simulink model "Appl_PaAdjustModel"  (R2018b)
settings: configuration reference "CodeConfig_10_ms" (kept outside this file)
undefined symbols (not defined in the file): CAL_HightMotorRunInterval_100ms, CAL_MotorDiffToStart_100ms, CAL_MotorStopTime_50ms, D_Relay_DownBackFault, D_Relay_UpFrontFault, D_ToleranceDistance, enSeatMoveCmd, FALSE, TRUE
libraries: DareLib x84, simulink x2
(part 2 of 3)

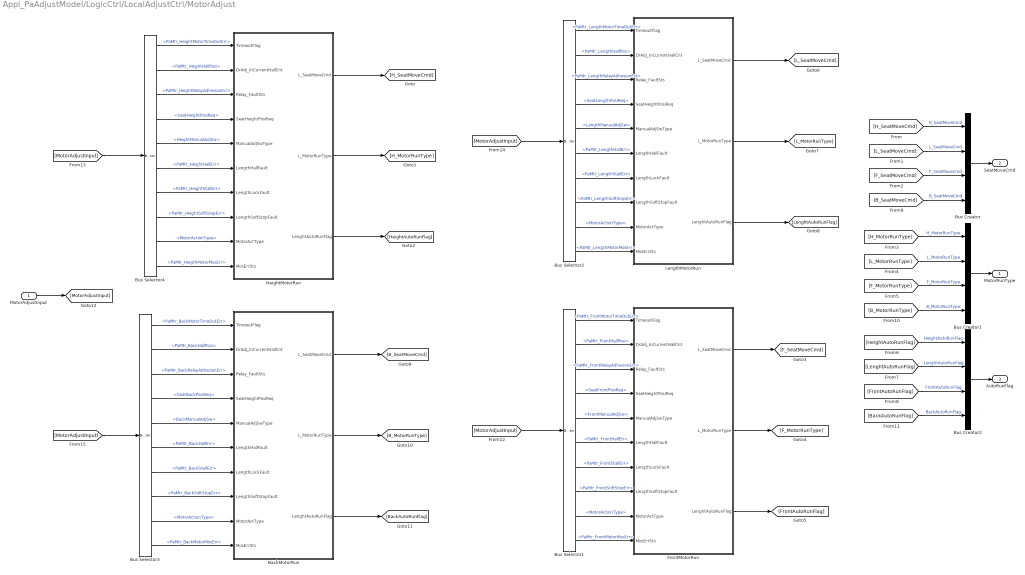
== system Appl_PaAdjustModel/LogicCtrl/LocalAdjustCtrl/MotorAdjust ==
  MotorAdjustInput : Inport
  BackMotorRun : Subsystem
      settings: AttributesFormatString=靠背电机运动状态与处理
  Bus Creator : BusCreator  Inputs=4
  Bus Creator1 : BusCreator  Inputs=4
  Bus Creator2 : BusCreator  Inputs=4
  Bus Selector1 : BusSelector  OutputSignals=RteInputBus.ErrSts.PaMtr_FrontMotorTimeOutErr,RteInputBus.HallCnt.PaMtr_FrontHallPosi,RteInputBus.ErrSts.PaMtr_FrontRelayAdhesionErr,MotorReq.SeatFrontPosiReq,MotorReq.FrontManualAdjSw,RteInputBus.ErrSts.PaMtr_FrontHallErr,RteInputBus.ErrSts.PaMtr_FrontStallErr,RteInputBus.ErrSts.PaMtr_FrontSoftStopErr,MotorReq.MotorActionType,RteInputBus.MosErrSts.PaMtr_FrontMotorMosErr
  Bus Selector2 : BusSelector  OutputSignals=RteInputBus.ErrSts.PaMtr_LengthMotorTimeOutErr,RteInputBus.HallCnt.PaMtr_LengthHallPosi,RteInputBus.ErrSts.PaMtr_LengthRelayAdhesionErr,MotorReq.SeatLengthPosiReq,MotorReq.LengthManualAdjSw,RteInputBus.ErrSts.PaMtr_LengthHallErr,RteInputBus.ErrSts.PaMtr_LengthStallErr,RteInputBus.ErrSts.PaMtr_LengthSoftStopErr,MotorReq.MotorActionType,RteInputBus.MosErrSts.PaMtr_LengthMotorMosErr
  Bus Selector3 : BusSelector  OutputSignals=RteInputBus.ErrSts.PaMtr_BackMotorTimeOutErr,RteInputBus.HallCnt.PaMtr_BackHallPosi,RteInputBus.ErrSts.PaMtr_BackRelayAdhesionErr,MotorReq.SeatBackPosiReq,MotorReq.BackManualAdjSw,RteInputBus.ErrSts.PaMtr_BackHallErr,RteInputBus.ErrSts.PaMtr_BackStallErr,RteInputBus.ErrSts.PaMtr_BackSoftStopErr,MotorReq.MotorActionType,RteInputBus.MosErrSts.PaMtr_BackMotorMosErr
  Bus Selector4 : BusSelector  OutputSignals=RteInputBus.ErrSts.PaMtr_HeightMotorTimeOutErr,RteInputBus.HallCnt.PaMtr_HeightHallPosi,RteInputBus.ErrSts.PaMtr_HeightRelayAdhesionErr,MotorReq.SeatHeightPosiReq,MotorReq.HeightManualAdjSw,RteInputBus.ErrSts.PaMtr_HeightHallErr,RteInputBus.ErrSts.PaMtr_HeightStallErr,RteInputBus.ErrSts.PaMtr_HeightSoftStopErr,MotorReq.MotorActionType,RteInputBus.MosErrSts.PaMtr_HeigthMotorMosErr
  FrontMotorRun : Subsystem
      settings: AttributesFormatString=腿托电机运动状态与处理
  HeightMotorRun : Subsystem
      settings: AttributesFormatString=高度电机运动状态与处理
  LengthMotorRun : Subsystem  Description=纵向电机
      settings: AttributesFormatString=纵向电机运动请求处理
  MotorRunType : Outport
  SeatMoveCmd : Outport  Port=2
  AutoRunFlag : Outport  Port=3
  wires:
  [H_SeatMoveCmd] -> Bus Creator/1  "H_SeatMoveCmd"
  [L_SeatMoveCmd] -> Bus Creator/2  "L_SeatMoveCmd"
  [F_SeatMoveCmd] -> Bus Creator/3  "F_SeatMoveCmd"
  [B_SeatMoveCmd] -> Bus Creator/4  "B_SeatMoveCmd"
  [H_MotorRunType] -> Bus Creator1/1  "H_MotorRunType"
  [L_MotorRunType] -> Bus Creator1/2  "L_MotorRunType"
  [F_MotorRunType] -> Bus Creator1/3  "F_MotorRunType"
  [B_MotorRunType] -> Bus Creator1/4  "B_MotorRunType"
  [LenghtAutoRunFlag] -> Bus Creator2/2  "LenghtAutoRunFlag"
  [HeightAutoRunFlag] -> Bus Creator2/1  "HeightAutoRunFlag"
  [FrontAutoRunFlag] -> Bus Creator2/3  "FrontAutoRunFlag"
  [BackAutoRunFlag] -> Bus Creator2/4  "BackAutoRunFlag"
  Bus Creator/1 -> SeatMoveCmd/1
  Bus Creator1/1 -> MotorRunType/1
  Bus Creator2/1 -> AutoRunFlag/1
  BackMotorRun/3(LenghtAutoRunFlag) -> [BackAutoRunFlag]
  LengthMotorRun/3(LenghtAutoRunFlag) -> [LenghtAutoRunFlag]
  FrontMotorRun/3(LenghtAutoRunFlag) -> [FrontAutoRunFlag]
  BackMotorRun/2(L_MotorRunType) -> [B_MotorRunType]
  LengthMotorRun/1(L_SeatMoveCmd) -> [L_SeatMoveCmd]
  FrontMotorRun/1(L_SeatMoveCmd) -> [F_SeatMoveCmd]
  HeightMotorRun/2(L_MotorRunType) -> [H_MotorRunType]
  LengthMotorRun/2(L_MotorRunType) -> [L_MotorRunType]
  HeightMotorRun/1(L_SeatMoveCmd) -> [H_SeatMoveCmd]
  HeightMotorRun/3(LenghtAutoRunFlag) -> [HeightAutoRunFlag]
  FrontMotorRun/2(L_MotorRunType) -> [F_MotorRunType]
  BackMotorRun/1(L_SeatMoveCmd) -> [B_SeatMoveCmd]
  MotorAdjustInput/1 -> [MotorAdjustInput]
  [MotorAdjustInput] -> Bus Selector4/1
  Bus Selector4/1 -> HeightMotorRun/1(TimeoutFlag)  "<PaMtr_HeightMotorTimeOutErr>"
  Bus Selector4/2 -> HeightMotorRun/2(DrAdj_InCurrentHallCnt)  "<PaMtr_HeightHallPosi>"
  Bus Selector4/3 -> HeightMotorRun/3(Relay_FaultSts)  "<PaMtr_HeightRelayAdhesionErr>"
  Bus Selector4/4 -> HeightMotorRun/4(SeatHeightPosiReq)  "<SeatHeightPosiReq>"
  Bus Selector4/5 -> HeightMotorRun/5(ManualAdjSwType)  "<HeightManualAdjSw>"
  Bus Selector4/6 -> HeightMotorRun/6(LengthHallFault)  "<PaMtr_HeightHallErr>"
  Bus Selector4/7 -> HeightMotorRun/7(LengthLockFault)  "<PaMtr_HeightStallErr>"
  Bus Selector4/8 -> HeightMotorRun/8(LengthSoftStopFault)  "<PaMtr_HeightSoftStopErr>"
  Bus Selector4/9 -> HeightMotorRun/9(MotorActType)  "<MotorActionType>"
  [MotorAdjustInput] -> Bus Selector2/1
  Bus Selector2/1 -> LengthMotorRun/1(TimeoutFlag)  "<PaMtr_LengthMotorTimeOutErr>"
  Bus Selector2/2 -> LengthMotorRun/2(DrAdj_InCurrentHallCnt)  "<PaMtr_LengthHallPosi>"
  Bus Selector2/3 -> LengthMotorRun/3(Relay_FaultSts)  "<PaMtr_LengthRelayAdhesionErr>"
  Bus Selector2/4 -> LengthMotorRun/4(SeatHeightPosiReq)  "<SeatLengthPosiReq>"
  Bus Selector2/5 -> LengthMotorRun/5(ManualAdjSwType)  "<LengthManualAdjSw>"
  Bus Selector2/6 -> LengthMotorRun/6(LengthHallFault)  "<PaMtr_LengthHallErr>"
  Bus Selector2/7 -> LengthMotorRun/7(LengthLockFault)  "<PaMtr_LengthStallErr>"
  Bus Selector2/8 -> LengthMotorRun/8(LengthSoftStopFault)  "<PaMtr_LengthSoftStopErr>"
  Bus Selector2/9 -> LengthMotorRun/9(MotorActType)  "<MotorActionType>"
  [MotorAdjustInput] -> Bus Selector3/1
  Bus Selector3/1 -> BackMotorRun/1(TimeoutFlag)  "<PaMtr_BackMotorTimeOutErr>"
  Bus Selector3/2 -> BackMotorRun/2(DrAdj_InCurrentHallCnt)  "<PaMtr_BackHallPosi>"
  Bus Selector3/3 -> BackMotorRun/3(Relay_FaultSts)  "<PaMtr_BackRelayAdhesionErr>"
  Bus Selector3/4 -> BackMotorRun/4(SeatHeightPosiReq)  "<SeatBackPosiReq>"
  Bus Selector3/5 -> BackMotorRun/5(ManualAdjSwType)  "<BackManualAdjSw>"
  Bus Selector3/6 -> BackMotorRun/6(LengthHallFault)  "<PaMtr_BackHallErr>"
  Bus Selector3/7 -> BackMotorRun/7(LengthLockFault)  "<PaMtr_BackStallErr>"
  Bus Selector3/8 -> BackMotorRun/8(LengthSoftStopFault)  "<PaMtr_BackSoftStopErr>"
  Bus Selector3/9 -> BackMotorRun/9(MotorActType)  "<MotorActionType>"
  [MotorAdjustInput] -> Bus Selector1/1
  Bus Selector1/1 -> FrontMotorRun/1(TimeoutFlag)  "<PaMtr_FrontMotorTimeOutErr>"
  Bus Selector1/2 -> FrontMotorRun/2(DrAdj_InCurrentHallCnt)  "<PaMtr_FrontHallPosi>"
  Bus Selector1/3 -> FrontMotorRun/3(Relay_FaultSts)  "<PaMtr_FrontRelayAdhesionErr>"
  Bus Selector1/4 -> FrontMotorRun/4(SeatHeightPosiReq)  "<SeatFrontPosiReq>"
  Bus Selector1/5 -> FrontMotorRun/5(ManualAdjSwType)  "<FrontManualAdjSw>"
  Bus Selector1/6 -> FrontMotorRun/6(LengthHallFault)  "<PaMtr_FrontHallErr>"
  Bus Selector1/7 -> FrontMotorRun/7(LengthLockFault)  "<PaMtr_FrontStallErr>"
  Bus Selector1/8 -> FrontMotorRun/8(LengthSoftStopFault)  "<PaMtr_FrontSoftStopErr>"
  Bus Selector1/9 -> FrontMotorRun/9(MotorActType)  "<MotorActionType>"
  Bus Selector1/10 -> FrontMotorRun/10(MosErrSts)  "<PaMtr_FrontMotorMosErr>"
  Bus Selector3/10 -> BackMotorRun/10(MosErrSts)  "<PaMtr_BackMotorMosErr>"
  Bus Selector2/10 -> LengthMotorRun/10(MosErrSts)  "<PaMtr_LengthMotorMosErr>"
  Bus Selector4/10 -> HeightMotorRun/10(MosErrSts)  "<PaMtr_HeigthMotorMosErr>"

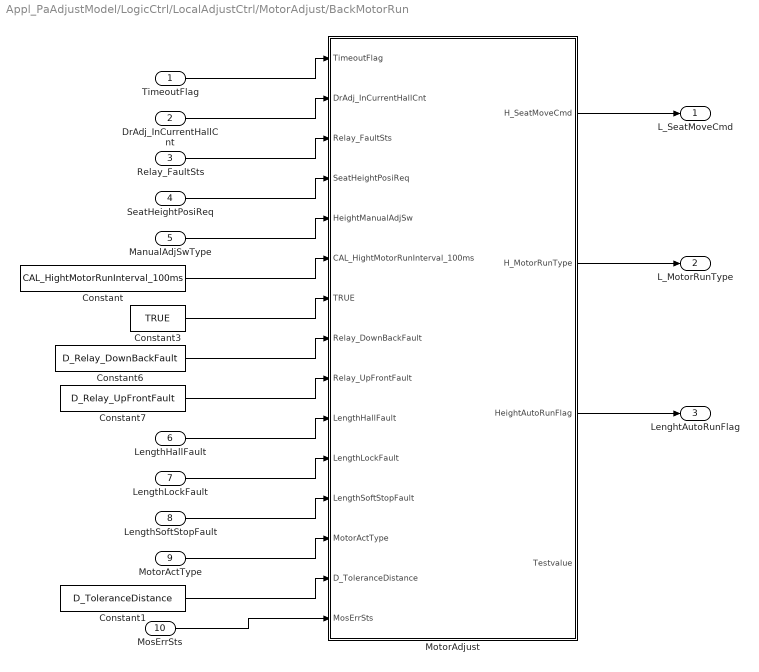
== system Appl_PaAdjustModel/LogicCtrl/LocalAdjustCtrl/MotorAdjust/BackMotorRun ==
  TimeoutFlag : Inport
  DrAdj_InCurrentHallCnt : Inport  Port=2
  Relay_FaultSts : Inport  Port=3
  SeatHeightPosiReq : Inport  Port=4
  ManualAdjSwType : Inport  Port=5
  LengthHallFault : Inport  Port=6
  LengthLockFault : Inport  Port=7
  LengthSoftStopFault : Inport  Port=8
  MotorActType : Inport  Port=9
  MosErrSts : Inport  Port=10
  Constant : Constant  Value=CAL_HightMotorRunInterval_100ms
  Constant1 : Constant  Value=D_ToleranceDistance
  Constant3 : Constant  Value=TRUE
  Constant6 : Constant  Value=D_Relay_DownBackFault
  Constant7 : Constant  Value=D_Relay_UpFrontFault
  MotorAdjust : Stateflow chart  TreatAsAtomicUnit=on
  L_SeatMoveCmd : Outport
  L_MotorRunType : Outport  Port=2
  LenghtAutoRunFlag : Outport  Port=3
  wires:
  Constant1/1 -> MotorAdjust/14(D_ToleranceDistance)
  MotorActType/1 -> MotorAdjust/13(MotorActType)
  LengthSoftStopFault/1 -> MotorAdjust/12(LengthSoftStopFault)
  LengthLockFault/1 -> MotorAdjust/11(LengthLockFault)
  LengthHallFault/1 -> MotorAdjust/10(LengthHallFault)
  TimeoutFlag/1 -> MotorAdjust/1(TimeoutFlag)
  Constant7/1 -> MotorAdjust/9(Relay_UpFrontFault)
  Constant6/1 -> MotorAdjust/8(Relay_DownBackFault)
  DrAdj_InCurrentHallCnt/1 -> MotorAdjust/2(DrAdj_InCurrentHallCnt)
  Relay_FaultSts/1 -> MotorAdjust/3(Relay_FaultSts)
  SeatHeightPosiReq/1 -> MotorAdjust/4(SeatHeightPosiReq)
  ManualAdjSwType/1 -> MotorAdjust/5(HeightManualAdjSw)
  MotorAdjust/1(H_SeatMoveCmd) -> L_SeatMoveCmd/1
  MotorAdjust/2(H_MotorRunType) -> L_MotorRunType/1
  MotorAdjust/3(HeightAutoRunFlag) -> LenghtAutoRunFlag/1
  Constant/1 -> MotorAdjust/6(CAL_HightMotorRunInterval_100ms)
  Constant3/1 -> MotorAdjust/7(TRUE)
  MosErrSts/1 -> MotorAdjust/15(MosErrSts)

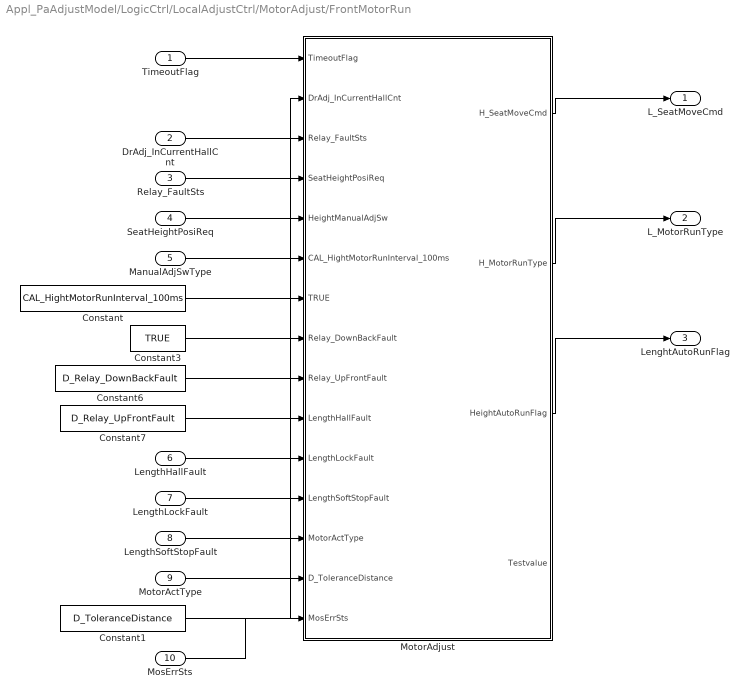
== system Appl_PaAdjustModel/LogicCtrl/LocalAdjustCtrl/MotorAdjust/FrontMotorRun ==
  TimeoutFlag : Inport
  DrAdj_InCurrentHallCnt : Inport  Port=2
  Relay_FaultSts : Inport  Port=3
  SeatHeightPosiReq : Inport  Port=4
  ManualAdjSwType : Inport  Port=5
  LengthHallFault : Inport  Port=6
  LengthLockFault : Inport  Port=7
  LengthSoftStopFault : Inport  Port=8
  MotorActType : Inport  Port=9
  MosErrSts : Inport  Port=10
  Constant : Constant  Value=CAL_HightMotorRunInterval_100ms
  Constant1 : Constant  Value=D_ToleranceDistance
  Constant3 : Constant  Value=TRUE
  Constant6 : Constant  Value=D_Relay_DownBackFault
  Constant7 : Constant  Value=D_Relay_UpFrontFault
  MotorAdjust : Stateflow chart  TreatAsAtomicUnit=on
  L_SeatMoveCmd : Outport
  L_MotorRunType : Outport  Port=2
  LenghtAutoRunFlag : Outport  Port=3
  wires:
  Constant3/1 -> MotorAdjust/7(TRUE)
  Constant/1 -> MotorAdjust/6(CAL_HightMotorRunInterval_100ms)
  MotorAdjust/3(HeightAutoRunFlag) -> LenghtAutoRunFlag/1
  MotorAdjust/2(H_MotorRunType) -> L_MotorRunType/1
  MotorAdjust/1(H_SeatMoveCmd) -> L_SeatMoveCmd/1
  ManualAdjSwType/1 -> MotorAdjust/5(HeightManualAdjSw)
  SeatHeightPosiReq/1 -> MotorAdjust/4(SeatHeightPosiReq)
  Relay_FaultSts/1 -> MotorAdjust/3(Relay_FaultSts)
  DrAdj_InCurrentHallCnt/1 -> MotorAdjust/2(DrAdj_InCurrentHallCnt)
  Constant6/1 -> MotorAdjust/8(Relay_DownBackFault)
  Constant7/1 -> MotorAdjust/9(Relay_UpFrontFault)
  TimeoutFlag/1 -> MotorAdjust/1(TimeoutFlag)
  LengthHallFault/1 -> MotorAdjust/10(LengthHallFault)
  LengthLockFault/1 -> MotorAdjust/11(LengthLockFault)
  LengthSoftStopFault/1 -> MotorAdjust/12(LengthSoftStopFault)
  MotorActType/1 -> MotorAdjust/13(MotorActType)
  Constant1/1 -> MotorAdjust/14(D_ToleranceDistance)
  MosErrSts/1 -> MotorAdjust/15(MosErrSts)

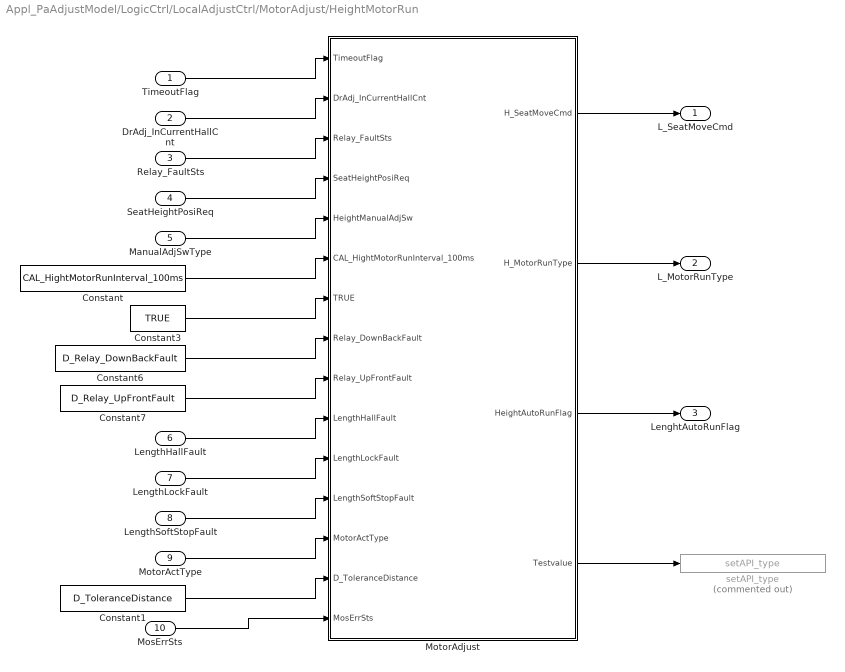
== system Appl_PaAdjustModel/LogicCtrl/LocalAdjustCtrl/MotorAdjust/HeightMotorRun ==
  TimeoutFlag : Inport
  DrAdj_InCurrentHallCnt : Inport  Port=2
  Relay_FaultSts : Inport  Port=3
  SeatHeightPosiReq : Inport  Port=4
  ManualAdjSwType : Inport  Port=5
  LengthHallFault : Inport  Port=6
  LengthLockFault : Inport  Port=7
  LengthSoftStopFault : Inport  Port=8
  MotorActType : Inport  Port=9
  MosErrSts : Inport  Port=10
  Constant : Constant  Value=CAL_HightMotorRunInterval_100ms
  Constant1 : Constant  Value=D_ToleranceDistance
  Constant3 : Constant  Value=TRUE
  Constant6 : Constant  Value=D_Relay_DownBackFault
  Constant7 : Constant  Value=D_Relay_UpFrontFault
  MotorAdjust : Stateflow chart  TreatAsAtomicUnit=on
  setAPI_type : DareLib/Dare/setAPI_type  Commented=on  g_funcname=Srvl_Set_D_SimuIndex_TestValue  g_param=D_SimuIndex_TestValue  g_type=uint8  g_size=-1
      settings: AttributesFormatString=%<g_funcname>  SourceProductName=Dare Library
  L_SeatMoveCmd : Outport
  L_MotorRunType : Outport  Port=2
  LenghtAutoRunFlag : Outport  Port=3
  wires:
  MotorAdjust/4(Testvalue) -> setAPI_type/1
  Constant1/1 -> MotorAdjust/14(D_ToleranceDistance)
  MotorActType/1 -> MotorAdjust/13(MotorActType)
  LengthSoftStopFault/1 -> MotorAdjust/12(LengthSoftStopFault)
  LengthLockFault/1 -> MotorAdjust/11(LengthLockFault)
  LengthHallFault/1 -> MotorAdjust/10(LengthHallFault)
  TimeoutFlag/1 -> MotorAdjust/1(TimeoutFlag)
  Constant7/1 -> MotorAdjust/9(Relay_UpFrontFault)
  Constant6/1 -> MotorAdjust/8(Relay_DownBackFault)
  DrAdj_InCurrentHallCnt/1 -> MotorAdjust/2(DrAdj_InCurrentHallCnt)
  Relay_FaultSts/1 -> MotorAdjust/3(Relay_FaultSts)
  SeatHeightPosiReq/1 -> MotorAdjust/4(SeatHeightPosiReq)
  ManualAdjSwType/1 -> MotorAdjust/5(HeightManualAdjSw)
  MotorAdjust/1(H_SeatMoveCmd) -> L_SeatMoveCmd/1
  MotorAdjust/2(H_MotorRunType) -> L_MotorRunType/1
  MotorAdjust/3(HeightAutoRunFlag) -> LenghtAutoRunFlag/1
  Constant/1 -> MotorAdjust/6(CAL_HightMotorRunInterval_100ms)
  Constant3/1 -> MotorAdjust/7(TRUE)
  MosErrSts/1 -> MotorAdjust/15(MosErrSts)

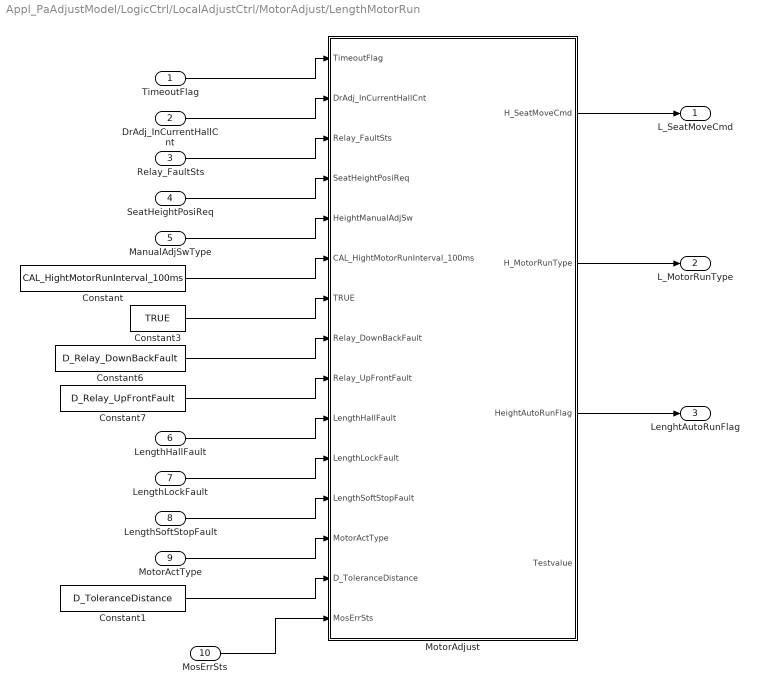
== system Appl_PaAdjustModel/LogicCtrl/LocalAdjustCtrl/MotorAdjust/LengthMotorRun ==
  TimeoutFlag : Inport
  DrAdj_InCurrentHallCnt : Inport  Port=2
  Relay_FaultSts : Inport  Port=3
  SeatHeightPosiReq : Inport  Port=4
  ManualAdjSwType : Inport  Port=5
  LengthHallFault : Inport  Port=6
  LengthLockFault : Inport  Port=7
  LengthSoftStopFault : Inport  Port=8
  MotorActType : Inport  Port=9
  MosErrSts : Inport  Port=10
  Constant : Constant  Value=CAL_HightMotorRunInterval_100ms
  Constant1 : Constant  Value=D_ToleranceDistance
  Constant3 : Constant  Value=TRUE
  Constant6 : Constant  Value=D_Relay_DownBackFault
  Constant7 : Constant  Value=D_Relay_UpFrontFault
  MotorAdjust : Stateflow chart  TreatAsAtomicUnit=on
  L_SeatMoveCmd : Outport
  L_MotorRunType : Outport  Port=2
  LenghtAutoRunFlag : Outport  Port=3
  wires:
  Constant3/1 -> MotorAdjust/7(TRUE)
  Constant/1 -> MotorAdjust/6(CAL_HightMotorRunInterval_100ms)
  MotorAdjust/3(HeightAutoRunFlag) -> LenghtAutoRunFlag/1
  MotorAdjust/2(H_MotorRunType) -> L_MotorRunType/1
  MotorAdjust/1(H_SeatMoveCmd) -> L_SeatMoveCmd/1
  ManualAdjSwType/1 -> MotorAdjust/5(HeightManualAdjSw)
  SeatHeightPosiReq/1 -> MotorAdjust/4(SeatHeightPosiReq)
  Relay_FaultSts/1 -> MotorAdjust/3(Relay_FaultSts)
  DrAdj_InCurrentHallCnt/1 -> MotorAdjust/2(DrAdj_InCurrentHallCnt)
  Constant6/1 -> MotorAdjust/8(Relay_DownBackFault)
  Constant7/1 -> MotorAdjust/9(Relay_UpFrontFault)
  TimeoutFlag/1 -> MotorAdjust/1(TimeoutFlag)
  LengthHallFault/1 -> MotorAdjust/10(LengthHallFault)
  LengthLockFault/1 -> MotorAdjust/11(LengthLockFault)
  LengthSoftStopFault/1 -> MotorAdjust/12(LengthSoftStopFault)
  MotorActType/1 -> MotorAdjust/13(MotorActType)
  Constant1/1 -> MotorAdjust/14(D_ToleranceDistance)
  MosErrSts/1 -> MotorAdjust/15(MosErrSts)

== stateflow chart Appl_PaAdjustModel/LogicCtrl/LocalAdjustCtrl/AdjustRequestPriority/PaMotorAdjustmentPriorityProcessing ==
  state MotorAdjPriorityPro
    en:
    TestValue2 = 0;
    du:
    TestValue2 = MotorActionType;
    note: 电机动作类型：
        | 0：无动作；
        | 1：HUM；
        | 2：舒适；
        | 3：记忆调用；
        | 4：手动调节；
        | 5：学习调节
        | 6：复位调节
        | 7：按摩调节
        | 8：小憩调节
    (default) -> (junction 85)
    MotorAdjPriorityPro -> (junction 85)
    (junction 85) -> (junction 236) : {
        | //无功能请求状态
        | MotorActionType = enSeatMotorRunTye.EN_NULL;
        | HeightManualAdjSw = 0;
        | LengthManualAdjSw = 0;
        | BackManualAdjSw = 0;
        | FrontManualAdjSw = 0;
        | SeatHeightPosiReq = 0;
        | SeatLengthPosiReq = 0;
        | SeatBackPosiReq = 0;
        | SeatFrontPosiReq = 0;
        | }
    (junction 236) -> (junction 238) [commented out] : [0 != HumSeatHeightPosi ...
        | || 0 != HumSeatLengthPosi ...
        | || 0 != HumSeatBackPosi...
        | || 0 != HumSeatFrontPosi]
    (junction 236) -> (junction 242)
    (junction 238) -> (junction 240) [commented out] : {
        | //档位请求有效
        | MotorActionType = enSeatMotorRunTye.EN_HUMEnable;
        | HeightManualAdjSw = 0;
        | LengthManualAdjSw = 0;
        | BackManualAdjSw = 0;
        | FrontManualAdjSw = 0;
        | SeatHeightPosiReq = HumSeatHeightPosi;
        | SeatLengthPosiReq = HumSeatLengthPosi;
        | SeatBackPosiReq = HumSeatBackPosi;
        | SeatFrontPosiReq = HumSeatFrontPosi;
        | }
    (junction 240) -> (junction 242) [commented out]
    (junction 242) -> (junction 306)
    (junction 306) -> (junction 308) [order 1] : [0 != PaMtr_WelcomeLengthReqPosi ...
        | || 0 != PaMtr_WelcomeBackReqPosi]
    (junction 306) -> (junction 312) [order 2]
    (junction 308) -> (junction 310) : {
        | //舒适调节请求有效
        | MotorActionType = enSeatMotorRunTye.EN_ComfortEnable;
        | HeightManualAdjSw = 0;
        | LengthManualAdjSw = 0;
        | BackManualAdjSw = 0;
        | FrontManualAdjSw = 0;
        | SeatHeightPosiReq = 0;
        | SeatLengthPosiReq = PaMtr_WelcomeLengthReqPosi;
        | SeatBackPosiReq = PaMtr_WelcomeBackReqPosi;
        | SeatFrontPosiReq = 0;
        | }
    (junction 310) -> (junction 312)
    (junction 312) -> (junction 315)
    (junction 315) -> (junction 319) [order 1] : [0 != PaMtr_MemoryHeightReqPosi ...
        | || 0 != PaMtr_MemoryLengthReqPosi ...
        | || 0 != PaMtr_MemoryBackReqPosi...
        | || 0 != PaMtr_MemoryFrontReqPosi]
    (junction 315) -> (junction 317) [order 2]
    (junction 319) -> (junction 321) : {
        | //记忆调节请求有效
        | MotorActionType = enSeatMotorRunTye.EN_MemoryEnable;
        | HeightManualAdjSw = 0;
        | LengthManualAdjSw = 0;
        | BackManualAdjSw = 0;
        | FrontManualAdjSw = 0;
        | SeatHeightPosiReq = PaMtr_MemoryHeightReqPosi;
        | SeatLengthPosiReq = PaMtr_MemoryLengthReqPosi;
        | SeatBackPosiReq = PaMtr_MemoryBackReqPosi;
        | SeatFrontPosiReq = PaMtr_MemoryFrontReqPosi;
        | }
    (junction 321) -> (junction 317)
    (junction 317) -> (junction 357)
    (junction 357) -> (junction 359) [commented out] : [0 != MtrCtrl_ResHeightReqPosi ...
        | || 0 != MtrCtrl_ResLengthReqPosi ...
        | || 0 != MtrCtrl_ResBackReqPosi...
        | || 0 != MtrCtrl_ResFrontReqPosi]
    (junction 357) -> (junction 363)
    (junction 359) -> (junction 361) [commented out] : {//小憩请求有效
        | MotorActionType = enSeatMotorRunTye.EN_ResEnable;
        | HeightManualAdjSw = 0;
        | LengthManualAdjSw = 0;
        | BackManualAdjSw = 0;
        | FrontManualAdjSw = 0;
        | SeatHeightPosiReq = MtrCtrl_ResHeightReqPosi;
        | SeatLengthPosiReq = MtrCtrl_ResLengthReqPosi;
        | SeatBackPosiReq = MtrCtrl_ResBackReqPosi;
        | SeatFrontPosiReq = MtrCtrl_ResFrontReqPosi;}
    (junction 361) -> (junction 363) [commented out]
    (junction 363) -> (junction 324)
    (junction 324) -> (junction 326) [order 1] : [(0 != PaMtr_ResetHeightReqPosi ...
        | || 0 != PaMtr_ResetLengthReqPosi...
        | || 0 != PaMtr_ResetBackReqPosi ...
        | || 0 != PaMtr_ResetFrontReqPosi)]
    (junction 324) -> (junction 332) [order 2]
    (junction 326) -> (junction 330) : {//复位调节有效
        | MotorActionType = enSeatMotorRunTye.EN_ResetEnable;
        | HeightManualAdjSw = 0;
        | LengthManualAdjSw = 0;
        | BackManualAdjSw = 0;
        | FrontManualAdjSw = 0;
        | SeatHeightPosiReq = PaMtr_ResetHeightReqPosi;
        | SeatLengthPosiReq = PaMtr_ResetLengthReqPosi;
        | SeatBackPosiReq = PaMtr_ResetBackReqPosi;
        | SeatFrontPosiReq = PaMtr_ResetFrontReqPosi;}
    (junction 330) -> (junction 332)
    (junction 332) -> (junction 335)
    (junction 335) -> (junction 337) [order 1] : [0 != PaMtr_HeightLearnCmd ...
        | || 0 != PaMtr_LengthLearnCmd ...
        | || 0 != PaMtr_BackLearnCmd ...
        | || 0 != PaMtr_FrontLearnCmd]
    (junction 335) -> (junction 341) [order 2]
    (junction 337) -> (junction 339) : {
        | //学习调节有效
        | MotorActionType = enSeatMotorRunTye.EN_LearnEnable;
        | HeightManualAdjSw = PaMtr_HeightLearnCmd;
        | LengthManualAdjSw = PaMtr_LengthLearnCmd;
        | BackManualAdjSw = PaMtr_BackLearnCmd;
        | FrontManualAdjSw = PaMtr_FrontLearnCmd;
        | SeatHeightPosiReq = 0;
        | SeatLengthPosiReq = 0;
        | SeatBackPosiReq = 0;
        | SeatFrontPosiReq = 0;
        | }
    (junction 339) -> (junction 341)
    (junction 341) -> (junction 344)
    (junction 344) -> (junction 346) [order 1] : [0 != PaMtr_HeightSwitchCmd ...
        | || 0 != PaMtr_LengthSwitchCmd ...
        | || 0 != PaMtr_BackSwitchCmd ...
        | || 0 != PaMtr_FrontSwitchCmd]
    (junction 344) -> (junction 350) [order 2]
    (junction 346) -> (junction 348) : {
        | //手动调节有效
        | MotorActionType = enSeatMotorRunTye.EN_ManualEnable;
        | HeightManualAdjSw = PaMtr_HeightSwitchCmd;
        | LengthManualAdjSw = PaMtr_LengthSwitchCmd;
        | BackManualAdjSw = PaMtr_BackSwitchCmd;
        | FrontManualAdjSw = PaMtr_FrontSwitchCmd;
        | SeatHeightPosiReq = 0;
        | SeatLengthPosiReq = 0;
        | SeatBackPosiReq = 0;
        | SeatFrontPosiReq = 0;
        | }
    (junction 348) -> (junction 350)
    (junction 350) -> (junction 355)
  (default) -> MotorAdjPriorityPro
  data: PaMtr_HeightSwitchCmd input; PaMtr_LengthSwitchCmd input; PaMtr_BackSwitchCmd input; MotorActionType output Enum: enSeatMotorRunTye; SeatHeightPosiReq output uint16; SeatLengthPosiReq output uint16; SeatBackPosiReq output uint16; SeatFrontPosiReq output uint16; HeightManualAdjSw output uint8; LengthManualAdjSw output uint8; BackManualAdjSw output uint8; FrontManualAdjSw output uint8; PaMtr_FrontSwitchCmd input; PaMtr_MemoryHeightReqPosi input; PaMtr_MemoryLengthReqPosi input; PaMtr_MemoryBackReqPosi input; TestValue2 output uint8; PaMtr_MemoryFrontReqPosi input; PaMtr_WelcomeLengthReqPosi input; PaMtr_WelcomeBackReqPosi input; PaMtr_HeightLearnCmd input; PaMtr_LengthLearnCmd input; PaMtr_BackLearnCmd input; PaMtr_FrontLearnCmd input; PaMtr_ResetHeightReqPosi input; PaMtr_ResetLengthReqPosi input; PaMtr_ResetBackReqPosi input; PaMtr_ResetFrontReqPosi input

== stateflow chart Appl_PaAdjustModel/LogicCtrl/LocalAdjustCtrl/MotorAdjust/HeightMotorRun/MotorAdjust ==
  note: 此处取霍尔值越往下越大约往后越大
  state Init_Interval
    en:
    H_SeatMoveCmd = enSeatMoveCmd.EN_NULL;
    HMotorRunIntervalTime = 1;
    DownBackFlag = 0;
    UpFrontFlag = 0;
    Testvalue = 1;
    du:
    ex:
    HMotorRunIntervalTime = 0;
    Init_Interval -> (junction 11) [order 1]
    (junction 11) -> (junction 13) [order 1] : /*高度电机调间隔时间*/
        | [HMotorRunIntervalTime < CAL_HightMotorRunInterval_100ms]
    (junction 11) -> (junction 17) [order 2]
    (junction 13) -> (junction 15) : {HMotorRunIntervalTime ++;}
    (junction 15) -> (junction 17)
    (junction 17) -> (junction 30) : {DownBackFlag = 0;
        | UpFrontFlag = 0;}
    (junction 30) -> (junction 32) [order 1] : /*高度自动调节有效*/
        | [0 != SeatHeightPosiReq]
    (junction 32) -> (junction 43) [order 1] : /*高度误差判断目前定义为5霍尔数值*/
        | [enSeatMoveCmd.EN_UP_FORWARD != LengthSoftStopFault ...
        | && SeatHeightPosiReq > DrAdj_InCurrentHallCnt ...
        | && D_ToleranceDistance < (SeatHeightPosiReq - DrAdj_InCurrentHallCnt)]
    (junction 30) -> (junction 39) [order 2] : { HeightAutoRunFlag = EN_SEAT_INVALID;}
    (junction 32) -> (junction 34) [order 2]
    (junction 43) -> (junction 45) : {UpFrontFlag = 1;}
    (junction 34) -> (junction 47) [order 1] : /* 不在软止点 且超误差范围 */
        | [enSeatMoveCmd.EN_DN_BACKWARD != LengthSoftStopFault ...
        | && SeatHeightPosiReq < DrAdj_InCurrentHallCnt ...
        | && D_ToleranceDistance < (DrAdj_InCurrentHallCnt - SeatHeightPosiReq)]
    (junction 34) -> (junction 52) [order 2] : /*高度误差范围内，反馈成功*/
        | {HeightAutoRunFlag = EN_SEAT_SUCCESS;
        | H_MotorRunType = EN_AutoAdjust_FUSuccess_Stop;}
    (junction 47) -> (junction 49) : {DownBackFlag = 1;}
    (junction 52) -> (junction 39)
    (junction 49) -> (junction 52)
    (junction 45) -> (junction 49)
    (junction 39) -> (junction 57)
    (junction 57) -> (junction 134)
    (junction 134) -> (junction 135) [order 1] : /* 调用位置有变化 则先清状态 */
        | [hasChanged(SeatHeightPosiReq)]
    (junction 134) -> (junction 133) [order 2]
    (junction 135) -> (junction 126) : {HeightAutoRunFlag = EN_SEAT_INVALID;}
    (junction 126) -> (junction 133)
    (junction 133) -> (junction 128)
  state H_MotorUpFrontRun
    en:
    H_SeatMoveCmd  = EN_UP_FORWARD
    Testvalue = 2;
    (default) -> (junction 64)
    H_MotorUpFrontRun -> (junction 64) [order 1]
    (junction 64) -> (junction 67) [order 1] : /*自动调节*/
        | [EN_AutoAdjust_FU == H_MotorRunType]
    (junction 64) -> (junction 71) [order 2] : {HeightAutoRunFlag = EN_SEAT_INVALID;}
    (junction 67) -> (junction 69) : {HeightAutoRunFlag = EN_SEAT_RUNNING;}
    (junction 69) -> (junction 71)
    (junction 71) -> (junction 74)
  state H_MotorDownBackRun
    en:
    H_SeatMoveCmd  = EN_DN_BACKWARD;
    Testvalue = 3;
    (default) -> (junction 87)
    H_MotorDownBackRun -> (junction 87) [order 1]
    (junction 87) -> (junction 81) [order 1] : /*高度自动调节*/
        | [EN_AutoAdjust_BK == H_MotorRunType]
    (junction 87) -> (junction 84) [order 2] : {HeightAutoRunFlag = EN_SEAT_INVALID;}
    (junction 81) -> (junction 77) : {HeightAutoRunFlag = EN_SEAT_RUNNING;}
    (junction 77) -> (junction 84)
    (junction 84) -> (junction 89)
  (default) -> Init_Interval
  Init_Interval -> H_MotorUpFrontRun [order 4] : /*高度继电器下后粘连故障 == 有效 间隔时间大于100ms*/
      | [Relay_DownBackFault ==  Relay_FaultSts...
      | && CAL_HightMotorRunInterval_100ms <= HMotorRunIntervalTime ]
      | /H_MotorRunType = EN_DnBkRelayAdhesion_FU;
  Init_Interval -> H_MotorDownBackRun [order 1] : /*高度继电器上前粘连故障 == 有效*/
      | [Relay_UpFrontFault == Relay_FaultSts ...
      | && CAL_HightMotorRunInterval_100ms <= HMotorRunIntervalTime ]
      | /H_MotorRunType = EN_DnFURelayAdhesion_BK;
  H_MotorUpFrontRun -> Init_Interval [order 3] : /*高度继电器下后粘连故障 != 有效*/
      | [Relay_DownBackFault != Relay_FaultSts...
      | && EN_DnBkRelayAdhesion_FU == H_MotorRunType]
      | /H_MotorRunType = EN_DnBkRelayAdhesion_FU_Stop;
  H_MotorDownBackRun -> Init_Interval [order 9] : /*高度继电器上前粘连故障 ！= 有效*/
      | [Relay_UpFrontFault != Relay_FaultSts  ...
      | && EN_DnFURelayAdhesion_BK == H_MotorRunType]
      | /H_MotorRunType = EN_DnFURelayAdhesion_BK_Stop;
  Init_Interval -> H_MotorUpFrontRun [order 3] : /*高度手动调节*/
      | [EN_UP_FORWARD == HeightManualAdjSw ...
      | && FALSE == LengthLockFault  ...
      | && FALSE == LengthHallFault ...
      | && FALSE == TimeoutFlag ...
      | && CAL_HightMotorRunInterval_100ms <= HMotorRunIntervalTime]
      | /H_MotorRunType = EN_ManualAdjust_FU;
  Init_Interval -> H_MotorDownBackRun [order 6] : /*高度手动调节有效*/
      | [EN_DN_BACKWARD == HeightManualAdjSw ...
      | && FALSE == LengthLockFault   ...
      | && FALSE == LengthHallFault...
      | && FALSE == TimeoutFlag ...
      | && CAL_HightMotorRunInterval_100ms <= HMotorRunIntervalTime]
      | /H_MotorRunType = EN_ManualAdjust_BK;
  H_MotorUpFrontRun -> Init_Interval [order 5] : /*高度手动调节无效*/
      | [(EN_UP_FORWARD != HeightManualAdjSw) ...
      | && EN_ManualAdjust_FU == H_MotorRunType]
      | /H_MotorRunType = EN_ManualAdjust_FU_Stop;
  H_MotorDownBackRun -> Init_Interval [order 7] : /*高度手动调节无效*/
      | [(EN_DN_BACKWARD != HeightManualAdjSw) ...
      | && EN_ManualAdjust_BK == H_MotorRunType]
      | /H_MotorRunType = EN_ManualAdjust_BK_Stop;
  Init_Interval -> H_MotorUpFrontRun [order 5] : /*高度自动调节有效且不在误差范围内*/
      | [0 != SeatHeightPosiReq ...
      | && FALSE == LengthLockFault ...
      | && HeightAutoRunFlag == EN_SEAT_INVALID ...
      | && UpFrontFlag == 1 ...
      | && CAL_HightMotorRunInterval_100ms <= HMotorRunIntervalTime]
      | /H_MotorRunType = EN_AutoAdjust_FU;
  Init_Interval -> H_MotorDownBackRun [order 2] : /*高度自动调节有效且不在误差范围内*/
      | [0 != SeatHeightPosiReq ...
      | && FALSE == LengthLockFault ...
      | && HeightAutoRunFlag == EN_SEAT_INVALID ...
      | && DownBackFlag == 1 ...
      | && CAL_HightMotorRunInterval_100ms <= HMotorRunIntervalTime]
      | /H_MotorRunType = EN_AutoAdjust_BK;
  H_MotorDownBackRun -> Init_Interval [order 3] : /*高度自动调节无效 设置电机运行类型BK停止 自动运行标志位失败*/
      | [0 == SeatHeightPosiReq ...
      | && EN_AutoAdjust_BK == H_MotorRunType]
      | /H_MotorRunType = EN_AutoAdjust_BK_Stop;
      | HeightAutoRunFlag =EN_SEAT_FAIL;
  H_MotorUpFrontRun -> Init_Interval [order 6] : /*高度自动调节无效 设置电机运行类型FU停止 自动运行标志位失败*/
      | [0 == SeatHeightPosiReq ...
      | && EN_AutoAdjust_FU == H_MotorRunType]
      | /H_MotorRunType = EN_AutoAdjust_FU_Stop;
      | HeightAutoRunFlag =EN_SEAT_FAIL
  H_MotorUpFrontRun -> Init_Interval [order 7] : /*高度自动调节成功 设置电机运行类型FU成功停止 自动运行标志位成功*/
      | [EN_AutoAdjust_FU == H_MotorRunType ...
      | && D_ToleranceDistance >= abs(SeatHeightPosiReq -  DrAdj_InCurrentHallCnt)]
      | /HeightAutoRunFlag = EN_SEAT_SUCCESS;
      | H_MotorRunType = EN_AutoAdjust_FUSuccess_Stop;
  H_MotorDownBackRun -> Init_Interval [order 4] : /*自动调节成功 设置电机运行类型成功停止 自动运行标志位成功*/
      | [EN_AutoAdjust_BK == H_MotorRunType ...
      | && D_ToleranceDistance >= abs(DrAdj_InCurrentHallCnt  - SeatHeightPosiReq)]
      | /HeightAutoRunFlag = EN_SEAT_SUCCESS;
      | H_MotorRunType = EN_AutoAdjust_BKSuccess_Stop;
  H_MotorUpFrontRun -> Init_Interval [order 9] : /*超时停止-非继电器粘连的驱动*/
      | [TRUE == TimeoutFlag ...
      | && Relay_DownBackFault !=  Relay_FaultSts]
      | /H_MotorRunType = EN_AutoAdjust_FUSuccess_Stop;
      | HeightAutoRunFlag =EN_SEAT_FAIL;
  H_MotorDownBackRun -> Init_Interval [order 8] : /*高度超时停止-非继电器粘连的驱动*/
      | [TRUE == TimeoutFlag ...
      | && Relay_UpFrontFault != Relay_FaultSts]
      | /H_MotorRunType = EN_AutoAdjust_BKSuccess_Stop;
      | HeightAutoRunFlag =EN_SEAT_FAIL;
  H_MotorUpFrontRun -> Init_Interval [order 4] : /* 高度向前到达止点，存在堵转故障，反馈成功 */
      | [/*FALSE == Relay_FaultSts &&*/ TRUE == LengthLockFault]
      | /H_MotorRunType = enSeatHightMotorRunsts.EN_UpFn_Lock_Stop;
      | HeightAutoRunFlag =EN_SEAT_SUCCESS;
  H_MotorDownBackRun -> Init_Interval [order 6] : /* 高度向后到达止点，存在堵转故障，反馈成功 */
      | [/*FALSE == Relay_FaultSts &&*/ TRUE == LengthLockFault]/
      | H_MotorRunType = enSeatHightMotorRunsts.EN_DnBa_Lock_Stop;
      | HeightAutoRunFlag =EN_SEAT_SUCCESS;
  H_MotorDownBackRun -> Init_Interval [order 10] : /* 存在霍尔故障 */
      | [/*FALSE == Relay_FaultSts &&*/ TRUE == LengthHallFault]
      | /H_MotorRunType = enSeatHightMotorRunsts.EN_DnBa_Hall_Stop;
      | HeightAutoRunFlag =EN_SEAT_FAIL;
  H_MotorUpFrontRun -> Init_Interval [order 10] : /* 高度存在霍尔故障 */
      | [/*FALSE == Relay_FaultSts && */TRUE == LengthHallFault]
      | /H_MotorRunType = enSeatHightMotorRunsts.EN_UpFn_Hall_Stop;
      | HeightAutoRunFlag =EN_SEAT_FAIL;
  H_MotorDownBackRun -> Init_Interval [order 11] : /* 存在MOS故障 */
      | [enMosErrSts.enNULL != MosErrSts]
      | /H_MotorRunType = enSeatHightMotorRunsts.EN_DnBa_MovTypeChange + MosErrSts;
      | HeightAutoRunFlag =EN_SEAT_FAIL;
  H_MotorUpFrontRun -> Init_Interval [order 11] : /* 高度存在MOS故障 */
      | [enMosErrSts.enNULL == MosErrSts]
      | /H_MotorRunType = enSeatHightMotorRunsts.EN_DnBa_MovTypeChange + MosErrSts;
      | HeightAutoRunFlag =EN_SEAT_FAIL;
  H_MotorDownBackRun -> Init_Interval [order 2] : /*自动调节-到达软止点停止 成功 */
      |  [EN_AutoAdjust_BK == H_MotorRunType ...
      | && enSeatMoveCmd.EN_DN_BACKWARD == LengthSoftStopFault]
      | /HeightAutoRunFlag = EN_SEAT_SUCCESS;
      | H_MotorRunType = EN_AutoAdjust_BKSuccess_Stop;
  H_MotorUpFrontRun -> Init_Interval [order 1] : /*自动调节-到达软止点停止 成功 */
      |  [EN_AutoAdjust_FU == H_MotorRunType ...
      | && enSeatMoveCmd.EN_UP_FORWARD == LengthSoftStopFault]
      | /HeightAutoRunFlag = EN_SEAT_SUCCESS;
      | H_MotorRunType = EN_AutoAdjust_FUSuccess_Stop;
  H_MotorDownBackRun -> Init_Interval [order 1] : /*高度控制类型改变
      | 优先级需要设定为1*/
      | [hasChanged(MotorActType)...
      |  && enSeatMotorRunTye.EN_NULL != MotorActType]
      | /HeightAutoRunFlag = EN_SEAT_INVALID;
      | H_MotorRunType = EN_DnBa_MovTypeChange;
  H_MotorUpFrontRun -> Init_Interval [order 2] : /*高度控制类型改变
      | 不能返回运动成功优先级需要设定为1*/
      | [hasChanged(MotorActType)...
      |  && enSeatMotorRunTye.EN_NULL != MotorActType]
      | /HeightAutoRunFlag = EN_SEAT_INVALID;
      | H_MotorRunType = EN_UpFn_MovTypeChange
  H_MotorDownBackRun -> Init_Interval [order 5] : /* 不在软止点 且超过误差范围，需要向前驱动 */
      | [0 != SeatHeightPosiReq ...
      | && SeatHeightPosiReq > DrAdj_InCurrentHallCnt]
      | /HeightAutoRunFlag = EN_SEAT_INVALID;
      | H_MotorRunType = EN_AutoAdjust_BK_Stop;
  H_MotorUpFrontRun -> Init_Interval [order 8] : /* 不在软止点 且超过误差范围，需要向后驱动 */
      | [0 != SeatHeightPosiReq ...
      | && SeatHeightPosiReq < DrAdj_InCurrentHallCnt]
      | /HeightAutoRunFlag = EN_SEAT_INVALID;
      | H_MotorRunType = EN_AutoAdjust_FU_Stop;
  data: TimeoutFlag input; DrAdj_InCurrentHallCnt input; Relay_FaultSts input; SeatHeightPosiReq input; HeightManualAdjSw input; H_SeatMoveCmd output Enum: enSeatMoveCmd; H_MotorRunType output Enum: enSeatHightMotorRunsts; CAL_HightMotorRunInterval_100ms input; DownBackFlag local uint8; UpFrontFlag local uint8; HeightAutoRunFlag output Enum: enSeatAutoRunSts; TRUE input; HMotorRunIntervalTime local uint8 =10; Relay_DownBackFault input; Relay_UpFrontFault input; LengthHallFault input; LengthLockFault input; FALSE parameter; LengthSoftStopFault input; MotorActType input; D_ToleranceDistance input; Testvalue output uint8; MosErrSts input Enum: enMosErrSts

== stateflow chart Appl_PaAdjustModel/LogicCtrl/LocalAdjustCtrl/FourMotorPriority/MotorMotionPriorityDeal ==
  note: 电机开启前后顺序遵循以下顺序：
      | 座椅高度＞座椅纵向＞座椅前部＞座椅靠背
  state HeightAdjust [parallel]
    settings: executionOrder=1
    state Action
      en:
      Hw_HeightMotorCtrl = HeightMotorCmd;
      Can_HeightMotorCtrl = HeightMotorCmd;
      du:
      Hw_HeightMotorCtrl = HeightMotorCmd;
      Can_HeightMotorCtrl = HeightMotorCmd;
      HeightTimer++;
      (default) -> (junction 487)
      HeightAdjust.Action -> (junction 487) [order 1]
      (junction 487) -> (junction 530) [order 1] : /* 继电器粘连*/
          | [FALSE != HeightRelayAdhesionErr]
      (junction 487) -> (junction 497) [order 2]
      (junction 530) -> (junction 488) : {HeightTimer = 0;}
      (junction 488) -> (junction 497)
      (junction 497) -> (junction 539)
    state Init
      en:
      Hw_HeightMotorCtrl = 0;
      Can_HeightMotorCtrl = 0;
      HeightTimer = 0;
    (default) -> HeightAdjust.Init
    HeightAdjust.Init -> HeightAdjust.Action : [EN_NULL != HeightMotorCmd]
    HeightAdjust.Action -> HeightAdjust.Init [order 1] : [EN_NULL == HeightMotorCmd]
  state VerticalAdjust [parallel]
    settings: executionOrder=2
    state Action
      en:
      Hw_LengthMotorCtrl = LengthMotorCmd;
      Can_LengthMotorCtrl = LengthMotorCmd;
      du:
      Hw_LengthMotorCtrl = LengthMotorCmd;
      Can_LengthMotorCtrl = LengthMotorCmd;
      LengthTimer++;
      (default) -> (junction 553)
      VerticalAdjust.Action -> (junction 553) [order 1]
      (junction 553) -> (junction 555) [order 1] : [FALSE != LengthRelayAdhesionErr]
      (junction 555) -> (junction 557) : {LengthTimer = 0;}
      (junction 553) -> (junction 554) [order 2]
      (junction 557) -> (junction 554)
      (junction 554) -> (junction 504)
    state Init
      en:
      Hw_LengthMotorCtrl = 0;
      Can_LengthMotorCtrl = 0;
      LengthTimer = 0;
    (default) -> VerticalAdjust.Init
    VerticalAdjust.Init -> VerticalAdjust.Action : /*高度、纵向电机没有命令或计时已到*/
        | [(EN_NULL == HeightMotorCmd || (EN_NULL != HeightMotorCmd && HeightTimer > CAL_MotorDiffToStart_100ms)) ...
        | && EN_NULL != LengthMotorCmd]
    VerticalAdjust.Action -> VerticalAdjust.Init [order 1] : [EN_NULL == LengthMotorCmd]
  state BackAdjust [parallel]
    settings: executionOrder=4
    state Action
      en:
      Hw_BackMotorCtrl = BackMotorCmd;
      Can_BackMotorCtrl = BackMotorCmd;
      du:
      Hw_BackMotorCtrl = BackMotorCmd;
      Can_BackMotorCtrl = BackMotorCmd;
      BackTimer++;
      (default) -> (junction 512)
      BackAdjust.Action -> (junction 512) [order 1]
      (junction 512) -> (junction 526) [order 1] : [FALSE != BackRelayAdhesionErr]
      (junction 512) -> (junction 542) [order 2]
      (junction 526) -> (junction 527) : {BackTimer = 0;}
      (junction 527) -> (junction 542)
      (junction 542) -> (junction 551)
    state Init
      en:
      Hw_BackMotorCtrl = 0;
      Can_BackMotorCtrl = 0;
      BackTimer = 0;
    (default) -> BackAdjust.Init
    BackAdjust.Init -> BackAdjust.Action : /*高度、纵向、前部电机没有命令或计时已到*/
        | [(EN_NULL == HeightMotorCmd || (EN_NULL != HeightMotorCmd && HeightTimer > CAL_MotorDiffToStart_100ms)) ...
        | && (EN_NULL == LengthMotorCmd || (EN_NULL != LengthMotorCmd && LengthTimer > CAL_MotorDiffToStart_100ms)) ...
        | && (EN_NULL == FrontMotorCmd || (EN_NULL != FrontMotorCmd && FrontTimer > CAL_MotorDiffToStart_100ms)) ...
        | && EN_NULL != BackMotorCmd]
    BackAdjust.Action -> BackAdjust.Init [order 1] : [EN_NULL == BackMotorCmd]
  state FrontAngleAdjust [parallel]
    settings: executionOrder=3
    state Action
      en:
      Hw_FrontMotorCtrl = FrontMotorCmd;
      Can_FrontMotorCtrl = FrontMotorCmd;
      du:
      Hw_FrontMotorCtrl = FrontMotorCmd;
      Can_FrontMotorCtrl = FrontMotorCmd;
      FrontTimer++;
      (default) -> (junction 519)
      FrontAngleAdjust.Action -> (junction 519) [order 1]
      (junction 519) -> (junction 485) [order 1] : [FALSE != FrontRelayAdhesionErr]
      (junction 519) -> (junction 529) [order 2]
      (junction 485) -> (junction 537) : {FrontTimer = 0;}
      (junction 537) -> (junction 529)
      (junction 529) -> (junction 524)
    state Init
      en:
      Hw_FrontMotorCtrl = 0;
      Can_FrontMotorCtrl = 0;
      FrontTimer = 0;
    (default) -> FrontAngleAdjust.Init
    FrontAngleAdjust.Init -> FrontAngleAdjust.Action : /*高度、纵向电机没有命令或计时已到*/
        | [(EN_NULL == HeightMotorCmd || (EN_NULL != HeightMotorCmd && HeightTimer > CAL_MotorDiffToStart_100ms)) ...
        | && (EN_NULL == LengthMotorCmd || (EN_NULL != LengthMotorCmd && LengthTimer > CAL_MotorDiffToStart_100ms)) ...
        | && EN_NULL != FrontMotorCmd]
    FrontAngleAdjust.Action -> FrontAngleAdjust.Init [order 1] : [EN_NULL == FrontMotorCmd]
  data: Can_HeightMotorCtrl output uint8; Can_LengthMotorCtrl output uint8; HeightMotorCmd input; LengthMotorCmd input; BackMotorCmd input; FrontMotorCmd input; EN_NULL input; CAL_MotorDiffToStart_100ms parameter; Can_BackMotorCtrl output uint8; Can_FrontMotorCtrl output uint8; FrontTimer local uint16; HeightTimer local uint16; LengthTimer local uint16; Hw_HeightMotorCtrl output uint8; Hw_LengthMotorCtrl output uint8; Hw_BackMotorCtrl output uint8; Hw_FrontMotorCtrl output uint8; BackTimer local uint16; HeightRelayAdhesionErr input; LengthRelayAdhesionErr input; BackRelayAdhesionErr input; FrontRelayAdhesionErr input; FALSE parameter

== stateflow chart Appl_PaAdjustModel/LogicCtrl/LocalAdjustCtrl/CrankAndVoltageDeal/CrankUnloading ==
  note: A.电源为CRANK
      | B.电压模式不满足
      | C.OTA模式
  state Init
    en:
    HeightMotorCmd = HeightMotorDirection;
    LengthMotorCmd = LengthMotorDirection;
    BackMotorCmd =  BackMotorDirection;
    FrontMotorCmd = FrontMotorDirection;
    du:
    HeightMotorCmd = HeightMotorDirection;
    LengthMotorCmd = LengthMotorDirection;
    BackMotorCmd = BackMotorDirection;
    FrontMotorCmd = FrontMotorDirection;
  state Ban
    //禁能
    en:
    HeightMotorCmd = 0;
    LengthMotorCmd = 0;
    BackMotorCmd = 0;
    FrontMotorCmd = 0;
  (default) -> Init
  Init -> Ban : /* 卸荷禁能 */
      | [enIgnSts.eCrank == PowerMode ...
      | || enFinalPowerMode.EN_NORMAL_VOLT != MtrCtrl_VoltMode || TRUE != MtrCtrl_VoltSatisfy...
      | || FALSE != DrAdj_OTABanFlag]
  Ban -> Init : /* 卸荷使能 */
      | [enIgnSts.eCrank != PowerMode ...
      | && enFinalPowerMode.EN_NORMAL_VOLT== MtrCtrl_VoltMode ...
      | && TRUE == MtrCtrl_VoltSatisfy ...
      | && FALSE == DrAdj_OTABanFlag]
  data: PowerMode input; MtrCtrl_VoltMode input; HeightMotorDirection input; LengthMotorDirection input; HeightMotorCmd output uint8; LengthMotorCmd output uint8; BackMotorDirection input; FrontMotorDirection input; BackMotorCmd output uint8; FrontMotorCmd output uint8; FALSE parameter; DrAdj_OTABanFlag input; MtrCtrl_VoltSatisfy input; TRUE parameter

== stateflow chart Appl_PaAdjustModel/LogicCtrl/LocalAdjustCtrl/MotorAdjust/LengthMotorRun/MotorAdjust ==
  note: 此处取霍尔值越往下越大约往后越大
  state Init_Interval
    en:
    H_SeatMoveCmd = enSeatMoveCmd.EN_NULL;
    HMotorRunIntervalTime = 1;
    DownBackFlag = 0;
    UpFrontFlag = 0;
    Testvalue = 1;
    du:
    ex:
    HMotorRunIntervalTime = 0;
    Init_Interval -> (junction 11) [order 1]
    (junction 11) -> (junction 13) [order 1] : /*纵向电机调间隔时间*/
        | [HMotorRunIntervalTime < CAL_HightMotorRunInterval_100ms]
    (junction 11) -> (junction 17) [order 2]
    (junction 13) -> (junction 15) : {HMotorRunIntervalTime ++;}
    (junction 15) -> (junction 17)
    (junction 17) -> (junction 30) : {DownBackFlag = 0;
        | UpFrontFlag = 0;}
    (junction 30) -> (junction 32) [order 1] : /*纵向自动调节有效*/
        | [0 != SeatHeightPosiReq]
    (junction 32) -> (junction 43) [order 1] : /*纵向误差判断目前定义为5霍尔数值*/
        | [enSeatMoveCmd.EN_UP_FORWARD != LengthSoftStopFault ...
        | && SeatHeightPosiReq > DrAdj_InCurrentHallCnt ...
        | && D_ToleranceDistance < (SeatHeightPosiReq - DrAdj_InCurrentHallCnt)]
    (junction 30) -> (junction 39) [order 2] : { HeightAutoRunFlag = EN_SEAT_INVALID;}
    (junction 32) -> (junction 34) [order 2]
    (junction 43) -> (junction 45) : {UpFrontFlag = 1;}
    (junction 34) -> (junction 47) [order 1] : /* 不在软止点 且超误差范围 */
        | [enSeatMoveCmd.EN_DN_BACKWARD != LengthSoftStopFault ...
        | && SeatHeightPosiReq < DrAdj_InCurrentHallCnt ...
        | && D_ToleranceDistance < (DrAdj_InCurrentHallCnt - SeatHeightPosiReq)]
    (junction 34) -> (junction 52) [order 2] : /*纵向误差范围内，反馈成功*/
        | {HeightAutoRunFlag = EN_SEAT_SUCCESS;
        | H_MotorRunType = EN_AutoAdjust_FUSuccess_Stop;}
    (junction 47) -> (junction 49) : {DownBackFlag = 1;}
    (junction 52) -> (junction 39)
    (junction 49) -> (junction 52)
    (junction 45) -> (junction 49)
    (junction 39) -> (junction 57)
    (junction 57) -> (junction 134)
    (junction 134) -> (junction 135) [order 1] : /* 调用位置有变化 则先清状态 */
        | [hasChanged(SeatHeightPosiReq)]
    (junction 134) -> (junction 133) [order 2]
    (junction 135) -> (junction 126) : {HeightAutoRunFlag = EN_SEAT_INVALID;}
    (junction 126) -> (junction 133)
    (junction 133) -> (junction 128)
  state H_MotorUpFrontRun
    en:
    H_SeatMoveCmd  = EN_UP_FORWARD
    Testvalue = 2;
    (default) -> (junction 64)
    H_MotorUpFrontRun -> (junction 64) [order 1]
    (junction 64) -> (junction 67) [order 1] : /*自动调节*/
        | [EN_AutoAdjust_FU == H_MotorRunType]
    (junction 64) -> (junction 71) [order 2] : {HeightAutoRunFlag = EN_SEAT_INVALID;}
    (junction 67) -> (junction 69) : {HeightAutoRunFlag = EN_SEAT_RUNNING;}
    (junction 69) -> (junction 71)
    (junction 71) -> (junction 74)
  state H_MotorDownBackRun
    en:
    H_SeatMoveCmd  = EN_DN_BACKWARD;
    Testvalue = 3;
    (default) -> (junction 87)
    H_MotorDownBackRun -> (junction 87) [order 1]
    (junction 87) -> (junction 81) [order 1] : /*纵向自动调节*/
        | [EN_AutoAdjust_BK == H_MotorRunType]
    (junction 87) -> (junction 84) [order 2] : {HeightAutoRunFlag = EN_SEAT_INVALID;}
    (junction 81) -> (junction 77) : {HeightAutoRunFlag = EN_SEAT_RUNNING;}
    (junction 77) -> (junction 84)
    (junction 84) -> (junction 89)
  (default) -> Init_Interval
  Init_Interval -> H_MotorUpFrontRun [order 4] : /*纵向继电器下后粘连故障 == 有效 间隔时间大于100ms*/
      | [Relay_DownBackFault ==  Relay_FaultSts...
      | && CAL_HightMotorRunInterval_100ms <= HMotorRunIntervalTime ]
      | /H_MotorRunType = EN_DnBkRelayAdhesion_FU;
  Init_Interval -> H_MotorDownBackRun [order 1] : /*纵向继电器上前粘连故障 == 有效*/
      | [Relay_UpFrontFault == Relay_FaultSts ...
      | && CAL_HightMotorRunInterval_100ms <= HMotorRunIntervalTime ]
      | /H_MotorRunType = EN_DnFURelayAdhesion_BK;
  H_MotorUpFrontRun -> Init_Interval [order 3] : /*纵向继电器下后粘连故障 != 有效*/
      | [Relay_DownBackFault != Relay_FaultSts...
      | && EN_DnBkRelayAdhesion_FU == H_MotorRunType]
      | /H_MotorRunType = EN_DnBkRelayAdhesion_FU_Stop;
  H_MotorDownBackRun -> Init_Interval [order 9] : /*纵向继电器上前粘连故障 ！= 有效*/
      | [Relay_UpFrontFault != Relay_FaultSts  ...
      | && EN_DnFURelayAdhesion_BK == H_MotorRunType]
      | /H_MotorRunType = EN_DnFURelayAdhesion_BK_Stop;
  Init_Interval -> H_MotorUpFrontRun [order 3] : /*纵向手动调节*/
      | [EN_UP_FORWARD == HeightManualAdjSw ...
      | && FALSE == LengthLockFault  ...
      | && FALSE == LengthHallFault ...
      | && FALSE == TimeoutFlag ...
      | && CAL_HightMotorRunInterval_100ms <= HMotorRunIntervalTime]
      | /H_MotorRunType = EN_ManualAdjust_FU;
  Init_Interval -> H_MotorDownBackRun [order 6] : /*纵向手动调节有效*/
      | [EN_DN_BACKWARD == HeightManualAdjSw ...
      | && FALSE == LengthLockFault   ...
      | && FALSE == LengthHallFault...
      | && FALSE == TimeoutFlag ...
      | && CAL_HightMotorRunInterval_100ms <= HMotorRunIntervalTime]
      | /H_MotorRunType = EN_ManualAdjust_BK;
  H_MotorUpFrontRun -> Init_Interval [order 5] : /*纵向手动调节无效*/
      | [(EN_UP_FORWARD != HeightManualAdjSw) ...
      | && EN_ManualAdjust_FU == H_MotorRunType]
      | /H_MotorRunType = EN_ManualAdjust_FU_Stop;
  H_MotorDownBackRun -> Init_Interval [order 7] : /*纵向手动调节无效*/
      | [(EN_DN_BACKWARD != HeightManualAdjSw) ...
      | && EN_ManualAdjust_BK == H_MotorRunType]
      | /H_MotorRunType = EN_ManualAdjust_BK_Stop;
  Init_Interval -> H_MotorUpFrontRun [order 5] : /*纵向自动调节有效且不在误差范围内*/
      | [0 != SeatHeightPosiReq ...
      | && FALSE == LengthLockFault ...
      | && HeightAutoRunFlag == EN_SEAT_INVALID ...
      | && UpFrontFlag == 1 ...
      | && CAL_HightMotorRunInterval_100ms <= HMotorRunIntervalTime]
      | /H_MotorRunType = EN_AutoAdjust_FU;
  Init_Interval -> H_MotorDownBackRun [order 2] : /*纵向自动调节有效且不在误差范围内*/
      | [0 != SeatHeightPosiReq ...
      | && FALSE == LengthLockFault ...
      | && HeightAutoRunFlag == EN_SEAT_INVALID ...
      | && DownBackFlag == 1 ...
      | && CAL_HightMotorRunInterval_100ms <= HMotorRunIntervalTime]
      | /H_MotorRunType = EN_AutoAdjust_BK;
  H_MotorDownBackRun -> Init_Interval [order 3] : /*纵向自动调节无效 设置电机运行类型BK停止 自动运行标志位失败*/
      | [0 == SeatHeightPosiReq ...
      | && EN_AutoAdjust_BK == H_MotorRunType]
      | /H_MotorRunType = EN_AutoAdjust_BK_Stop;
      | HeightAutoRunFlag =EN_SEAT_FAIL;
  H_MotorUpFrontRun -> Init_Interval [order 6] : /*纵向自动调节无效 设置电机运行类型FU停止 自动运行标志位失败*/
      | [0 == SeatHeightPosiReq ...
      | && EN_AutoAdjust_FU == H_MotorRunType]
      | /H_MotorRunType = EN_AutoAdjust_FU_Stop;
      | HeightAutoRunFlag =EN_SEAT_FAIL
  H_MotorUpFrontRun -> Init_Interval [order 7] : /*纵向自动调节成功 设置电机运行类型FU成功停止 自动运行标志位成功*/
      | [EN_AutoAdjust_FU == H_MotorRunType ...
      | && D_ToleranceDistance >= abs(SeatHeightPosiReq -  DrAdj_InCurrentHallCnt)]
      | /HeightAutoRunFlag = EN_SEAT_SUCCESS;
      | H_MotorRunType = EN_AutoAdjust_FUSuccess_Stop;
  H_MotorDownBackRun -> Init_Interval [order 4] : /*自动调节成功 设置电机运行类型成功停止 自动运行标志位成功*/
      | [EN_AutoAdjust_BK == H_MotorRunType ...
      | && D_ToleranceDistance >= abs(DrAdj_InCurrentHallCnt  - SeatHeightPosiReq)]
      | /HeightAutoRunFlag = EN_SEAT_SUCCESS;
      | H_MotorRunType = EN_AutoAdjust_BKSuccess_Stop;
  H_MotorUpFrontRun -> Init_Interval [order 9] : /*纵向超时停止-非继电器粘连的驱动*/
      | [TRUE == TimeoutFlag ...
      | && Relay_DownBackFault !=  Relay_FaultSts]
      | /H_MotorRunType = EN_AutoAdjust_FUSuccess_Stop;
      | HeightAutoRunFlag =EN_SEAT_FAIL;
  H_MotorDownBackRun -> Init_Interval [order 8] : /*纵向超时停止-非继电器粘连的驱动*/
      | [TRUE == TimeoutFlag ...
      | && Relay_UpFrontFault != Relay_FaultSts]
      | /H_MotorRunType = EN_AutoAdjust_BKSuccess_Stop;
      | HeightAutoRunFlag =EN_SEAT_FAIL;
  H_MotorUpFrontRun -> Init_Interval [order 4] : /* 纵向向前到达止点，存在堵转故障，反馈成功 */
      | [/*FALSE == Relay_FaultSts &&*/ TRUE == LengthLockFault]
      | /H_MotorRunType = enSeatHightMotorRunsts.EN_UpFn_Lock_Stop;
      | HeightAutoRunFlag =EN_SEAT_SUCCESS;
  H_MotorDownBackRun -> Init_Interval [order 6] : /* 纵向向后到达止点，存在堵转故障，反馈成功 */
      | [/*FALSE == Relay_FaultSts &&*/ TRUE == LengthLockFault]/
      | H_MotorRunType = enSeatHightMotorRunsts.EN_DnBa_Lock_Stop;
      | HeightAutoRunFlag =EN_SEAT_SUCCESS;
  H_MotorUpFrontRun -> Init_Interval [order 10] : /* 纵向存在霍尔故障 */
      | [/*FALSE == Relay_FaultSts && */TRUE == LengthHallFault]
      | /H_MotorRunType = enSeatHightMotorRunsts.EN_UpFn_Hall_Stop;
      | HeightAutoRunFlag =EN_SEAT_FAIL;
  H_MotorDownBackRun -> Init_Interval [order 11] : /* 存在霍尔故障 */
      | [/*FALSE == Relay_FaultSts &&*/ TRUE == LengthHallFault]
      | /H_MotorRunType = enSeatHightMotorRunsts.EN_DnBa_Hall_Stop;
      | HeightAutoRunFlag =EN_SEAT_FAIL;
  H_MotorDownBackRun -> Init_Interval [order 10] : /* 存在MOS故障 */
      | [enMosErrSts.enNULL != MosErrSts]
      | /H_MotorRunType = enSeatHightMotorRunsts.EN_DnBa_MovTypeChange + MosErrSts;
      | HeightAutoRunFlag =EN_SEAT_FAIL;
  H_MotorUpFrontRun -> Init_Interval [order 11] : /* 纵向存在MOS故障 */
      | [enMosErrSts.enNULL != MosErrSts]
      | /H_MotorRunType = enSeatHightMotorRunsts.EN_DnBa_MovTypeChange + MosErrSts;
      | HeightAutoRunFlag =EN_SEAT_FAIL;
  H_MotorDownBackRun -> Init_Interval [order 2] : /*自动调节-到达软止点停止 成功 */
      |  [EN_AutoAdjust_BK == H_MotorRunType ...
      | && enSeatMoveCmd.EN_DN_BACKWARD == LengthSoftStopFault]
      | /HeightAutoRunFlag = EN_SEAT_SUCCESS;
      | H_MotorRunType = EN_AutoAdjust_BKSuccess_Stop;
  H_MotorUpFrontRun -> Init_Interval [order 1] : /*自动调节-到达软止点停止 成功 */
      |  [EN_AutoAdjust_FU == H_MotorRunType ...
      | && enSeatMoveCmd.EN_UP_FORWARD == LengthSoftStopFault]
      | /HeightAutoRunFlag = EN_SEAT_SUCCESS;
      | H_MotorRunType = EN_AutoAdjust_FUSuccess_Stop;
  H_MotorDownBackRun -> Init_Interval [order 1] : /*纵向控制类型改变
      | 优先级需要设定为1*/
      | [hasChanged(MotorActType)...
      |  && enSeatMotorRunTye.EN_NULL != MotorActType]
      | /HeightAutoRunFlag = EN_SEAT_INVALID;
      | H_MotorRunType = EN_DnBa_MovTypeChange;
  H_MotorUpFrontRun -> Init_Interval [order 2] : /*纵向控制类型改变
      | 不能返回运动成功优先级需要设定为1*/
      | [hasChanged(MotorActType)...
      |  && enSeatMotorRunTye.EN_NULL != MotorActType]
      | /HeightAutoRunFlag = EN_SEAT_INVALID;
      | H_MotorRunType = EN_UpFn_MovTypeChange
  H_MotorDownBackRun -> Init_Interval [order 5] : /* 不在软止点 且超过误差范围，需要向前驱动 */
      | [0 != SeatHeightPosiReq ...
      | && SeatHeightPosiReq > DrAdj_InCurrentHallCnt]
      | /HeightAutoRunFlag = EN_SEAT_INVALID;
      | H_MotorRunType = EN_AutoAdjust_BK_Stop;
  H_MotorUpFrontRun -> Init_Interval [order 8] : /* 不在软止点 且超过误差范围，需要向后驱动 */
      | [0 != SeatHeightPosiReq ...
      | && SeatHeightPosiReq < DrAdj_InCurrentHallCnt]
      | /HeightAutoRunFlag = EN_SEAT_INVALID;
      | H_MotorRunType = EN_AutoAdjust_FU_Stop;
  data: TimeoutFlag input; DrAdj_InCurrentHallCnt input; Relay_FaultSts input; SeatHeightPosiReq input; HeightManualAdjSw input; H_SeatMoveCmd output Enum: enSeatMoveCmd; H_MotorRunType output Enum: enSeatHightMotorRunsts; CAL_HightMotorRunInterval_100ms input; DownBackFlag local uint8; UpFrontFlag local uint8; HeightAutoRunFlag output Enum: enSeatAutoRunSts; TRUE input; HMotorRunIntervalTime local uint8 =10; Relay_DownBackFault input; Relay_UpFrontFault input; LengthHallFault input; LengthLockFault input; FALSE parameter; LengthSoftStopFault input; MotorActType input; D_ToleranceDistance input; Testvalue output uint8; MosErrSts input Enum: enMosErrSts
